simulink model "control"  (R2020a)
settings: Solver=ode3  StartTime=0.0  StopTime=10.0  MaxStep=0.02  RelTol=1e-3
libraries: roblocks x3
settings Model: Creator=robot  LastModifiedBy=robot

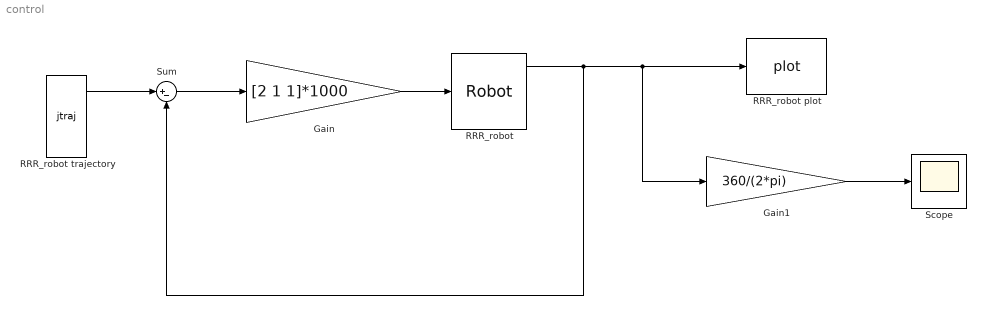
== system control ==
  Gain : Gain  Gain=[2 1 1]*1000
  Gain1 : Gain  Gain=360/(2*pi)
  RRR_robot : roblocks/Arm/Robot  robot=RRR_robot  q0=[0 0 0]
  RRR_robot plot : roblocks/Arm/plot  robot=RRR_robot  fps=5  holdplot=on
  RRR_robot trajectory : roblocks/Toolbox/jtraj  q0=[0 0 0]  qf=[pi/2 -pi/4 -pi/4]  tmax=2  ts=0.02
  Scope : Scope
  Sum : Sum  Inputs=|+-
  wires:
  RRR_robot trajectory/1 -> Sum/1
  Sum/1 -> Gain/1
  Gain/1 -> RRR_robot/1
  RRR_robot/1 -> Gain1/1, RRR_robot plot/1, Sum/2
  Gain1/1 -> Scope/1
